simulink model "LQG_Discrete"  (R2021b)
settings: Solver=VariableStepAuto  StartTime=0.0  StopTime=10  RelTol=1e-3
values from neighbouring files (symbols this model uses):
  Fd = lqrd(A,B,Q,R,1e-3)    [simConstants.m]
  sys2d = c2d(sys2,Ts)    [simConstants.m]
  Td = 100e-6    (= 0.0001)    [simConstants.m]
  Ts = 1e-3    (= 0.001)    [simConstants.m]
undefined symbols (not defined in the file or in its folder): Ld
libraries: simulink_extras x1
settings Model: Creator=logan  LastModifiedBy=logan

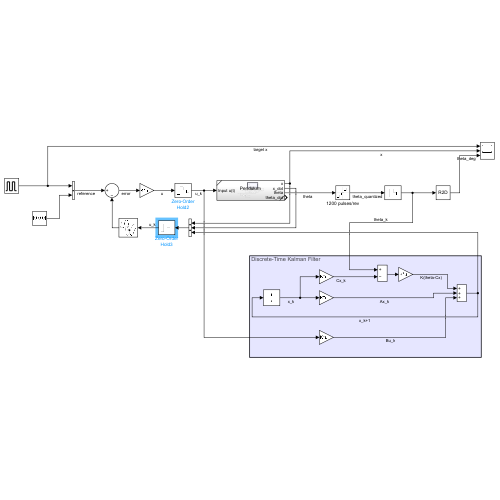
[thumbnail: Simulink's stored preview of the top-level diagram]
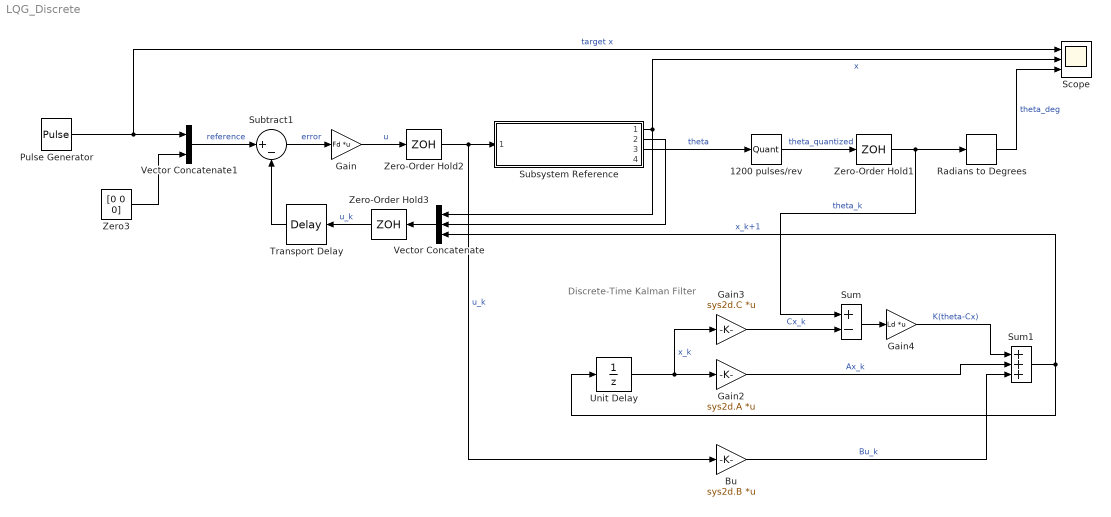
== system LQG_Discrete ==
  note: Discrete-Time Kalman Filter
  1200 pulses/rev : Quantizer  QuantizationInterval=(2*pi)/1200
  Bu : Gain  Gain=sys2d.B  Multiplication=Matrix(K*u)
  Gain : Gain  Gain=Fd  Multiplication=Matrix(K*u)
  Gain2 : Gain  Gain=sys2d.A  Multiplication=Matrix(K*u)
  Gain3 : Gain  Gain=sys2d.C  Multiplication=Matrix(K*u)
  Gain4 : Gain  Gain=Ld  Multiplication=Matrix(K*u)
  Pulse Generator : DiscretePulseGenerator  PulseType=Time based  Amplitude=0.5  Period=20  PulseWidth=50
  Radians to Degrees : simulink_extras/Transformations/Radians to Degrees
  Scope : Scope  NumInputPorts=3
  Subsystem Reference : Subsystem  ReferencedSubsystem=Pendulum
  Subtract1 : Sum  Inputs=|+-
  Sum : Sum  Inputs=+-
  Sum1 : Sum  Inputs=+++
  Transport Delay : TransportDelay  DelayTime=Td*10  InitialOutput=[0 0 0 0]
  Unit Delay : UnitDelay  SampleTime=Ts  HasFrameUpgradeWarning=on
  Vector Concatenate : Concatenate  NumInputs=3
  Vector Concatenate1 : Concatenate
  Zero-Order Hold1 : ZeroOrderHold  SampleTime=Ts
  Zero-Order Hold2 : ZeroOrderHold  SampleTime=Ts
  Zero-Order Hold3 : ZeroOrderHold  SampleTime=Ts
  Zero3 : Constant  Value=[0 0 0]  OutDataTypeStr=Inherit: Inherit via back propagation
  wires:
  Subtract1/1 -> Gain/1  "error"
  Subsystem Reference/3 -> 1200 pulses/rev/1  "theta"
  Subsystem Reference/1 -> Scope/2, Vector Concatenate/1  "x"
  Subsystem Reference/2 -> Vector Concatenate/2
  Radians to Degrees/1 -> Scope/3  "theta_deg"
  Zero3/1 -> Vector Concatenate1/2
  Vector Concatenate1/1 -> Subtract1/1  "reference"
  Pulse Generator/1 -> Scope/1, Vector Concatenate1/1  "target x"
  Vector Concatenate/1 -> Zero-Order Hold3/1
  Transport Delay/1 -> Subtract1/2
  Zero-Order Hold2/1 -> Bu/1, Subsystem Reference/1  "u_k"
  Gain2/1 -> Sum1/2  "Ax_k"
  Zero-Order Hold1/1 -> Sum/1, Radians to Degrees/1  "theta_k"
  Unit Delay/1 -> Gain3/1, Gain2/1  "x_k"
  Bu/1 -> Sum1/3  "Bu_k"
  Sum/1 -> Gain4/1
  Gain4/1 -> Sum1/1  "K(theta-Cx)"
  Gain3/1 -> Sum/2  "Cx_k"
  Gain/1 -> Zero-Order Hold2/1  "u"
  Sum1/1 -> Vector Concatenate/3, Unit Delay/1  "x_k+1"
  1200 pulses/rev/1 -> Zero-Order Hold1/1  "theta_quantized"
  Zero-Order Hold3/1 -> Transport Delay/1  "u_k"
